simulink model "sixDoFDynamics_th"  (R2018b)
settings: Solver=VariableStepAuto  StartTime=0.0  StopTime=10.0  RelTol=1e-3
values from neighbouring files (symbols this model uses):
  FNetBdy = [0;0;-1000]    [sixDoFDynamics_ts.m]
  MI = eye(3)    [sixDoFDynamics_ts.m]
  MNetBdy = [0;0;0]    [sixDoFDynamics_ts.m]
libraries: sixDoFDynamics_ul x1
settings Model: Creator=asiddiq2  LastModifiedBy=asiddiq2

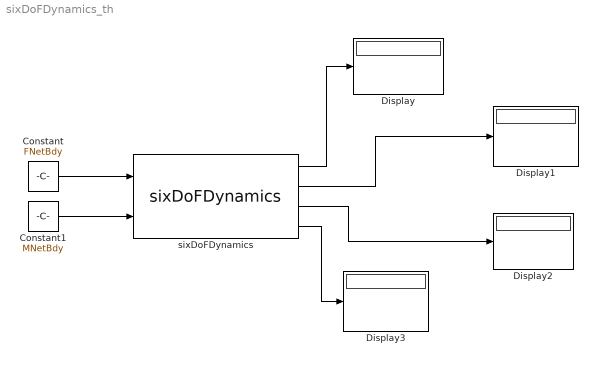
== system sixDoFDynamics_th ==
  Constant : Constant  Value=FNetBdy
  Constant1 : Constant  Value=MNetBdy
  Display{,1..3} (4 alike) : Display
  sixDoFDynamics : sixDoFDynamics_ul/sixDoFDynamics  M=mass_mat  initPos=ini_pos  initVel=ini_vel  J=MI  initEulAngs=ini_eul  initAngVel=ini_OwB
  wires:
  sixDoFDynamics/1 -> Display/1
  sixDoFDynamics/4 -> Display3/1
  sixDoFDynamics/3 -> Display2/1
  sixDoFDynamics/2 -> Display1/1
  Constant/1 -> sixDoFDynamics/1
  Constant1/1 -> sixDoFDynamics/2
